simulink model "Randomized_Blending_kalman_filters"  (R2018a)
settings: Solver=ode45  StartTime=0.0  StopTime=35  FixedStep=0.05  MaxStep=0.06  RelTol=1e-3  EnableMultiTasking=on
model workspace (MAT data in the model file):
  MCOS : class17 (value not decoded)
undefined symbols (not defined in the file or in its folder): altitude_error, Continuous, error1, error2, error3, error4, fault_time, IC, quadModel, Time
libraries: simulink x5, ctrlSharedLib x4
(part 2 of 2)

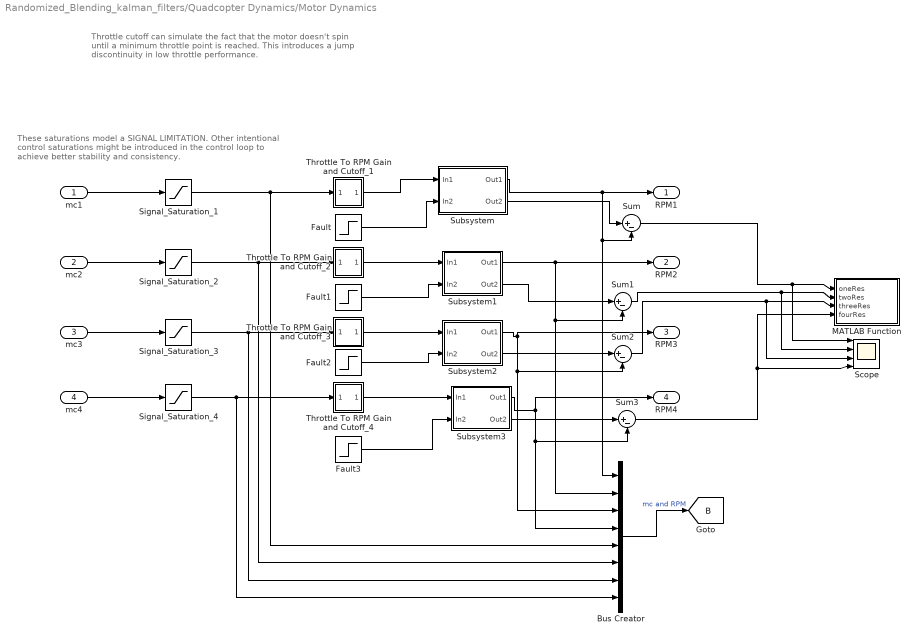
== system Randomized_Blending_kalman_filters/Quadcopter Dynamics/Motor Dynamics ==
  note: Throttle cutoff can simulate the fact that the motor doesn't
      | spin until a minimum throttle point is reached. This introduces
      | a jump discontinuity in low throttle performance.
  note: These saturations model a SIGNAL LIMITATION.
      | Other intentional control saturations might be introduced in the
      | control loop to achieve better stability and consistency.
  mc1 : Inport
  mc2 : Inport  Port=2
  mc3 : Inport  Port=3
  mc4 : Inport  Port=4
  Bus Creator : BusCreator  Inputs=8
  Fault : Step  Time=fault_time  After=error1  SampleTime=0
  Fault1 : Step  Time=fault_time  After=error2  SampleTime=0
  Fault2 : Step  Time=fault_time  After=error3  SampleTime=0
  Fault3 : Step  Time=fault_time  After=error4  SampleTime=0
  MATLAB Function : MATLAB Function  TreatAsAtomicUnit=on
  Scope : Scope  NumInputPorts=4
  Signal_Saturation_{1..4} (4 alike) : Saturate  UpperLimit=100  LowerLimit=0
  Subsystem : Subsystem
  Subsystem1 : Subsystem
  Subsystem2 : Subsystem
  Subsystem3 : Subsystem
  Sum{,1..3} (4 alike) : Sum  Inputs=|+-
  Throttle To RPM Gain and Cutoff_1 : Subsystem
  Throttle To RPM Gain and Cutoff_2 : Subsystem
  Throttle To RPM Gain and Cutoff_3 : Subsystem
  Throttle To RPM Gain and Cutoff_4 : Subsystem
  RPM1 : Outport
  RPM2 : Outport  Port=2
  RPM3 : Outport  Port=3
  RPM4 : Outport  Port=4
  tag scope: B=global
  wires:
  mc1/1 -> Signal_Saturation_1/1
  mc4/1 -> Signal_Saturation_4/1
  mc2/1 -> Signal_Saturation_2/1
  mc3/1 -> Signal_Saturation_3/1
  Signal_Saturation_1/1 -> Bus Creator/5, Throttle To RPM Gain and Cutoff_1/1(In5)
  Signal_Saturation_2/1 -> Bus Creator/6, Throttle To RPM Gain and Cutoff_2/1(In5)
  Signal_Saturation_3/1 -> Bus Creator/7, Throttle To RPM Gain and Cutoff_3/1(In5)
  Signal_Saturation_4/1 -> Bus Creator/8, Throttle To RPM Gain and Cutoff_4/1(In5)
  Throttle To RPM Gain and Cutoff_4/1(Out5) -> Subsystem3/1(In1)
  Subsystem3/1(Out1) -> RPM4/1, Sum3/2, Bus Creator/4
  Bus Creator/1 -> [B]  "mc and RPM"
  Subsystem/1(Out1) -> Sum/2, Bus Creator/1, RPM1/1
  Throttle To RPM Gain and Cutoff_1/1(Out5) -> Subsystem/1(In1)
  Fault/1 -> Subsystem/2(In2)
  Subsystem2/1(Out1) -> Sum2/2, Bus Creator/3, RPM3/1
  Subsystem1/1(Out1) -> Sum1/2, Bus Creator/2, RPM2/1
  Throttle To RPM Gain and Cutoff_2/1(Out5) -> Subsystem1/1(In1)
  Throttle To RPM Gain and Cutoff_3/1(Out5) -> Subsystem2/1(In1)
  Fault2/1 -> Subsystem2/2(In2)
  Fault3/1 -> Subsystem3/2(In2)
  Fault1/1 -> Subsystem1/2(In2)
  Subsystem/2(Out2) -> Sum/1
  Sum/1 -> Scope/1, MATLAB Function/1(oneRes)
  Subsystem3/2(Out2) -> Sum3/1
  Subsystem2/2(Out2) -> Sum2/1
  Subsystem1/2(Out2) -> Sum1/1
  Sum3/1 -> Scope/4, MATLAB Function/4(fourRes)
  Sum2/1 -> Scope/3, MATLAB Function/3(threeRes)
  Sum1/1 -> Scope/2, MATLAB Function/2(twoRes)

== system Randomized_Blending_kalman_filters/Quadcopter Dynamics/Motor Dynamics/Subsystem ==
  note: kalman filter
  note: Multiplicitive Fault
  In1 : Inport
  In2 : Inport  Port=2
  Kalman Filter : ctrlSharedLib/Kalman Filter  TimeDomain=Continuous-Time  UseCurrentEstimator=on  ModelSource=Individual A, B, C, D matrices  ModelSourceVariable=quadcopterDynamicsSFunction  A=-1/quadModel.T  B=1  C=1/quadModel.T  D=0  NumberOfStates=1  NumberOfInputs=1  NumberOfOutputs=1  InitialEstimateSource=Dialog  X0=0  P0=10  UseK=off  UseGH=off  NumberOfProcessNoiseInputs=1  G=1  TimeInvariantG=on  H=0  TimeInvariantH=on  Q=0.05  TimeInvariantQ=on  R=1  TimeInvariantR=on  N=0  TimeInvariantN=on  AddInputPort=on  AddEnablePort=off  OutputEstimatedY=on  OutputP=off  Ts=-1
      settings: SourceProductBaseCode=CT
  MATLAB Function : MATLAB Function  TreatAsAtomicUnit=on
  Motor_Dynamics_1 : StateSpace  A=-1/quadModel.T  C=1/quadModel.T  D=0  InitialCondition=IC.w1*quadModel.T
  Scope : Scope
  Out1 : Outport
  Out2 : Outport  Port=2
  wires:
  In1/1 -> Kalman Filter/1, Motor_Dynamics_1/1
  MATLAB Function/1(rotor_speed) -> Out1/1, Kalman Filter/2
  In2/1 -> MATLAB Function/1(fault)
  Motor_Dynamics_1/1 -> MATLAB Function/2(nominal_model_input)
  Kalman Filter/2 -> Scope/1, Out2/1

== system Randomized_Blending_kalman_filters/Quadcopter Dynamics/Motor Dynamics/Subsystem1 ==
  In1 : Inport
  In2 : Inport  Port=2
  Kalman Filter : ctrlSharedLib/Kalman Filter  TimeDomain=Continuous-Time  UseCurrentEstimator=on  ModelSource=Individual A, B, C, D matrices  ModelSourceVariable=quadcopterDynamicsSFunction  A=-1/quadModel.T  B=1  C=1/quadModel.T  D=0  NumberOfStates=1  NumberOfInputs=1  NumberOfOutputs=1  InitialEstimateSource=Dialog  X0=0  P0=10  UseK=off  UseGH=off  NumberOfProcessNoiseInputs=1  G=1  TimeInvariantG=on  H=0  TimeInvariantH=on  Q=0.05  TimeInvariantQ=on  R=1  TimeInvariantR=on  N=0  TimeInvariantN=on  AddInputPort=on  AddEnablePort=off  OutputEstimatedY=on  OutputP=off  Ts=-1
      settings: SourceProductBaseCode=CT
  MATLAB Function : MATLAB Function  TreatAsAtomicUnit=on
  "Motor_Dynamics_2 " : StateSpace  A=-1/quadModel.T  C=1/quadModel.T  D=0  InitialCondition=IC.w1*quadModel.T
  Out1 : Outport
  Out2 : Outport  Port=2
  wires:
  In1/1 -> "Motor_Dynamics_2 "/1, Kalman Filter/1
  MATLAB Function/1(rotor_speed) -> Kalman Filter/2, Out1/1
  In2/1 -> MATLAB Function/1(fault)
  "Motor_Dynamics_2 "/1 -> MATLAB Function/2(nominal_modal_input)
  Kalman Filter/2 -> Out2/1

== system Randomized_Blending_kalman_filters/Quadcopter Dynamics/Motor Dynamics/Subsystem2 ==
  In1 : Inport
  In2 : Inport  Port=2
  Kalman Filter : ctrlSharedLib/Kalman Filter  TimeDomain=Continuous-Time  UseCurrentEstimator=on  ModelSource=Individual A, B, C, D matrices  ModelSourceVariable=quadcopterDynamicsSFunction  A=-1/quadModel.T  B=1  C=1/quadModel.T  D=0  NumberOfStates=1  NumberOfInputs=1  NumberOfOutputs=1  InitialEstimateSource=Dialog  X0=0  P0=10  UseK=off  UseGH=off  NumberOfProcessNoiseInputs=1  G=1  TimeInvariantG=on  H=0  TimeInvariantH=on  Q=0.05  TimeInvariantQ=on  R=1  TimeInvariantR=on  N=0  TimeInvariantN=on  AddInputPort=on  AddEnablePort=off  OutputEstimatedY=on  OutputP=off  Ts=-1
      settings: SourceProductBaseCode=CT
  MATLAB Function : MATLAB Function  TreatAsAtomicUnit=on
  "Motor_Dynamics_3 " : StateSpace  A=-1/quadModel.T  C=1/quadModel.T  D=0  InitialCondition=IC.w1*quadModel.T
  Out1 : Outport
  Out2 : Outport  Port=2
  wires:
  In1/1 -> "Motor_Dynamics_3 "/1, Kalman Filter/1
  MATLAB Function/1(rotor_speed) -> Kalman Filter/2, Out1/1
  In2/1 -> MATLAB Function/1(fault)
  "Motor_Dynamics_3 "/1 -> MATLAB Function/2(nominal_modal_input)
  Kalman Filter/2 -> Out2/1

== system Randomized_Blending_kalman_filters/Quadcopter Dynamics/Motor Dynamics/Subsystem3 ==
  In1 : Inport
  In2 : Inport  Port=2
  Kalman Filter : ctrlSharedLib/Kalman Filter  TimeDomain=Continuous-Time  UseCurrentEstimator=on  ModelSource=Individual A, B, C, D matrices  ModelSourceVariable=quadcopterDynamicsSFunction  A=-1/quadModel.T  B=1  C=1/quadModel.T  D=0  NumberOfStates=1  NumberOfInputs=1  NumberOfOutputs=1  InitialEstimateSource=Dialog  X0=0  P0=10  UseK=off  UseGH=off  NumberOfProcessNoiseInputs=1  G=1  TimeInvariantG=on  H=0  TimeInvariantH=on  Q=0.05  TimeInvariantQ=on  R=1  TimeInvariantR=on  N=0  TimeInvariantN=on  AddInputPort=on  AddEnablePort=off  OutputEstimatedY=on  OutputP=off  Ts=-1
      settings: SourceProductBaseCode=CT
  MATLAB Function : MATLAB Function  TreatAsAtomicUnit=on
  "Motor_Dynamics_4 " : StateSpace  A=-1/quadModel.T  C=1/quadModel.T  D=0  InitialCondition=IC.w1*quadModel.T
  Out1 : Outport
  Out2 : Outport  Port=2
  wires:
  In1/1 -> Kalman Filter/1, "Motor_Dynamics_4 "/1
  MATLAB Function/1(rotor_speed) -> Kalman Filter/2, Out1/1
  In2/1 -> MATLAB Function/1(fault)
  "Motor_Dynamics_4 "/1 -> MATLAB Function/2(nominal_modal_input)
  Kalman Filter/2 -> Out2/1

== system Randomized_Blending_kalman_filters/Quadcopter Dynamics/Motor Dynamics/Throttle To RPM Gain and Cutoff_1 ==
  note: minThr should be a quad.mat value
  note: This gain should be a quad.mat value
  note: This constant should be a quad.mat value
  note: Output equals linearly scaled RPM
      | for given throttle input if throttle input >=Throttle Cuttoff (minThr)
      | else output is zero.
  In5 : Inport
  Constant : Constant  Value=quadModel.b
  Gain : Gain  Gain=quadModel.cr
  Minimum Throttle Cutoff : simulink/Logic and Bit Operations/Compare To Constant  relop=>=  const=quadModel.minThr  OutDataTypeStr=uint8
  Product : Product
  Sum1 : Sum  Inputs=++|
  Out5 : Outport
  wires:
  Minimum Throttle Cutoff/1 -> Product/2
  Product/1 -> Out5/1
  In5/1 -> Gain/1, Minimum Throttle Cutoff/1
  Gain/1 -> Sum1/2
  Sum1/1 -> Product/1
  Constant/1 -> Sum1/1

== system Randomized_Blending_kalman_filters/Quadcopter Dynamics/Motor Dynamics/Throttle To RPM Gain and Cutoff_2 ==
  note: minThr should be a quad.mat value
  note: This gain should be a quad.mat value
  note: This constant should be a quad.mat value
  note: Output equals linearly scaled RPM
      | for given throttle input if throttle input >=Throttle Cuttoff (minThr)
      | else output is zero.
  In5 : Inport
  Constant : Constant  Value=quadModel.b
  Gain : Gain  Gain=quadModel.cr
  Minimum Throttle Cutoff : simulink/Logic and Bit Operations/Compare To Constant  relop=>=  const=quadModel.minThr  OutDataTypeStr=uint8
  Product : Product
  Sum1 : Sum  Inputs=++|
  Out5 : Outport
  wires:
  Minimum Throttle Cutoff/1 -> Product/2
  Product/1 -> Out5/1
  In5/1 -> Gain/1, Minimum Throttle Cutoff/1
  Gain/1 -> Sum1/2
  Sum1/1 -> Product/1
  Constant/1 -> Sum1/1

== system Randomized_Blending_kalman_filters/Quadcopter Dynamics/Motor Dynamics/Throttle To RPM Gain and Cutoff_3 ==
  note: minThr should be a quad.mat value
  note: This gain should be a quad.mat value
  note: This constant should be a quad.mat value
  note: Output equals linearly scaled RPM
      | for given throttle input if throttle input >=Throttle Cuttoff (minThr)
      | else output is zero.
  In5 : Inport
  Constant : Constant  Value=quadModel.b
  Gain : Gain  Gain=quadModel.cr
  Minimum Throttle Cutoff : simulink/Logic and Bit Operations/Compare To Constant  relop=>=  const=quadModel.minThr  OutDataTypeStr=uint8
  Product : Product
  Sum1 : Sum  Inputs=++|
  Out5 : Outport
  wires:
  Minimum Throttle Cutoff/1 -> Product/2
  Product/1 -> Out5/1
  In5/1 -> Gain/1, Minimum Throttle Cutoff/1
  Gain/1 -> Sum1/2
  Sum1/1 -> Product/1
  Constant/1 -> Sum1/1

== system Randomized_Blending_kalman_filters/Quadcopter Dynamics/Motor Dynamics/Throttle To RPM Gain and Cutoff_4 ==
  note: minThr should be a quad.mat value
  note: This gain should be a quad.mat value
  note: This constant should be a quad.mat value
  note: Output equals linearly scaled RPM
      | for given throttle input if throttle input >=Throttle Cuttoff (minThr)
      | else output is zero.
  In5 : Inport
  Constant : Constant  Value=quadModel.b
  Gain : Gain  Gain=quadModel.cr
  Minimum Throttle Cutoff : simulink/Logic and Bit Operations/Compare To Constant  relop=>=  const=quadModel.minThr  OutDataTypeStr=uint8
  Product : Product
  Sum1 : Sum  Inputs=++|
  Out5 : Outport
  wires:
  Minimum Throttle Cutoff/1 -> Product/2
  Product/1 -> Out5/1
  In5/1 -> Gain/1, Minimum Throttle Cutoff/1
  Gain/1 -> Sum1/2
  Sum1/1 -> Product/1
  Constant/1 -> Sum1/1

== matlab function Randomized_Blending_kalman_filters/Quadcopter Dynamics/Motor Dynamics/Subsystem/MATLAB Function ==
  data: fault input; nominal_model_input input; rotor_speed output
function rotor_speed = fcn(fault, nominal_model_input)

rotor_speed =(nominal_model_input* (1-fault));

end

== matlab function Randomized_Blending_kalman_filters/Attitude Controller/blending  ==
  data: mode input; control_signal output; portion input; fault_controller input; nominal_controller input; wind_controller input
function control_signal = blending(mode , portion , fault_controller, nominal_controller, wind_controller)


if(mode == 1)
    fault_part = (fault_controller * portion);
    nominal_portion = 1-portion;
    nominal_part = nominal_controller * nominal_portion;
    control_signal = fault_part + nominal_part;
elseif(mode == 2)
    wind_part = (wind_controller * portion);
    nominal_portion = 1-portion;
    nominal_part = nominal_controller * nominal_portion;
    control_signal = wind_part + nominal_part;
elseif(mode == 3)
    fault_part = (fault_controller * (portion/2));
    nominal_portion = 1-portion;
    wind_part = wind_controller * (portion/2);
    nominal_part = nominal_controller * nominal_portion;
    control_signal = nominal_part + wind_part + fault_part;
else
    control_signal = nominal_controller;
end

== matlab function Randomized_Blending_kalman_filters/Quadcopter Dynamics/Motor Dynamics/Subsystem1/MATLAB Function ==
  data: fault input; nominal_modal_input input; rotor_speed output
function rotor_speed = fcn(  fault, nominal_modal_input)


rotor_speed =  (nominal_modal_input* (1-fault));

end

== matlab function Randomized_Blending_kalman_filters/Position Controller/MATLAB Function ==
  settings: updateMethod=DISCRETE
  data: y_error input; x_error input; max_error_signal data_store_memory; count data_store_memory; time input; prevTime data_store_memory
function fcn(y_error,x_error,time)
global prevTime;
global max_error_signal;
global count;
%if(abs(y_error) + abs(x_error) > max_error_signal)
if(prevTime+0.1 < time)
    max_error_signal = max_error_signal + abs(y_error) + abs(x_error);
    count =count +1;
    %disp(count);
    prevTime = time;
end
end

== matlab function Randomized_Blending_kalman_filters/Quadcopter Dynamics/Motor Dynamics/Subsystem2/MATLAB Function ==
  data: fault input; nominal_modal_input input; rotor_speed output
function rotor_speed = fcn(  fault, nominal_modal_input)


rotor_speed =  (nominal_modal_input* (1-fault));

end

== matlab function Randomized_Blending_kalman_filters/Quadcopter Dynamics/Motor Dynamics/Subsystem3/MATLAB Function ==
  data: fault input; nominal_modal_input input; rotor_speed output
function rotor_speed = fcn(  fault, nominal_modal_input)


rotor_speed =  (nominal_modal_input* (1-fault));

end

== matlab function Randomized_Blending_kalman_filters/Attitude Controller/blending 1 ==
  data: mode input; control_signal output; portion input; fault_controller input; nominal_controller input; wind_controller input
function control_signal = blending(mode , portion , fault_controller, nominal_controller, wind_controller)


if(mode == 1)
    fault_part = (fault_controller * portion);
    nominal_portion = 1-portion;
    nominal_part = nominal_controller * nominal_portion;
    control_signal = fault_part + nominal_part;
elseif(mode == 2)
    wind_part = (wind_controller * portion);
    nominal_portion = 1-portion;
    nominal_part = nominal_controller * nominal_portion;
    control_signal = wind_part + nominal_part;
elseif(mode == 3)
    fault_part = (fault_controller * (portion/2));
    nominal_portion = 1-portion;
    wind_part = wind_controller * (portion/2);
    nominal_part = nominal_controller * nominal_portion;
    control_signal = nominal_part + wind_part + fault_part;
else
    control_signal = nominal_controller;
end

== matlab function Randomized_Blending_kalman_filters/Attitude Controller/blending 2 ==
  data: mode input; control_signal output; portion input; fault_controller input; nominal_controller input; wind_controller input
function control_signal = blending(mode , portion , fault_controller, nominal_controller, wind_controller)


if(mode == 1)
    fault_part = (fault_controller * portion);
    nominal_portion = 1-portion;
    nominal_part = nominal_controller * nominal_portion;
    control_signal = fault_part + nominal_part;
elseif(mode == 2)
    wind_part = (wind_controller * portion);
    nominal_portion = 1-portion;
    nominal_part = nominal_controller * nominal_portion;
    control_signal = wind_part + nominal_part;
elseif(mode == 3)
    fault_part = (fault_controller * (portion/2));
    nominal_portion = 1-portion;
    wind_part = wind_controller * (portion/2);
    nominal_part = nominal_controller * nominal_portion;
    control_signal = nominal_part + wind_part + fault_part;
else
    control_signal = nominal_controller;
end

== matlab function Randomized_Blending_kalman_filters/Attitude Controller/High Level Randomised Algorithm ==
  settings: updateMethod=DISCRETE
  data: x_error input; y_error input; Phi output; Theta output; Psi output; previousTime data_store_memory; blend data_store_memory; time input; Phi_blend data_store_memory; Theta_blend data_store_memory; Psi_blend data_store_memory; errors data_store_memory; rate_of_change data_store_memory; rate output; current_error output; prev_rate_of_change data_store_memory; fault_est data_store_memory; fault output
function [Phi, Theta, Psi, rate, current_error, fault] = fcn(x_error, y_error, time)
%global lookup_table;
global previousTime;
global errors;
%current_error_index = (current_error*1000) +1;
global Phi_blend;
global Theta_blend;
global Psi_blend;
global rate_of_change;
global prev_rate_of_change;

global fault_est;

%distance to desired location
current_error = sqrt(x_error^2 + y_error^2);

%previous distance and current distance
if(time > previousTime(5))
    errors(1) = errors(2);
    errors(2) = errors(3);
    errors(3) = errors(4);
    errors(4) = errors(5);
    errors(5) = current_error;

    previousTime(1) = previousTime(2);
    previousTime(2) = previousTime(3);
    previousTime(3) = previousTime(4);
    previousTime(4) = previousTime(5);
    previousTime(5) = time;

    curve = polyfit(previousTime,errors , 4);
    derivative = polyder(curve);
    prev_rate_of_change = rate_of_change;
    rate_of_change =  polyval(derivative,time);
    %disp('--------------');
    %disp(time);
    %disp(rate_of_change);
    %disp(abs(current_error));
    rate = rate_of_change;
    
else
    rate = rate_of_change;
end
%if(rate_of_change > 0.3 && prev_rate_of_change > 0.3 && current_error > 0.3)

if(time > 15 )
    %blend = 0;
    %blend = 1;
    %blend = rand();
    %Phi = blend;
    %Theta= blend;
    %Psi = blend;
    %(BOTH WIND AND ROTOR)
    %fault = 3;
    % Phi_blend = blend;
    %Theta_blend =blend;
    %Psi_blend = blend;
    Phi = Phi_blend;
    Theta= Theta_blend;
    Psi = Psi_blend;
    fault = 1;
    
%no rotor fault but external disturbance 
elseif( time > 17 && rate_of_change > 0.2 && prev_rate_of_change > 0.2 )
    blend = rand();
    Phi = blend;
    Theta= blend;
    Psi = blend;
    fault = 1;
    %blend = 1;
    %
    %blend = 0;
    %Phi = blend;
    %Theta= blend;
    %Psi = blend;
    %(WIND)
    %fault = 2;
    %Phi_blend = blend;
    %Theta_blend =blend;
    %Psi_blend = blend;

%rotor fault and external disturbance
%elseif(fault_est == 1)
    %blend = rand();
    %blend = 1;
   % blend = 0;
   % Phi = blend;
   % Theta= blend;
    %Psi = blend;
    %(ROTOR)
    %fault = 1;
   % Phi_blend = blend;
    %Theta_blend =blend;
    %Psi_blend = blend;
    %Phi = Phi_blend;
    %Theta= Theta_blend;
    %Psi = Psi_blend;
    %fault = 1;
else
    %(No fault)
    blend = 0;
    %Phi = blend;
    %Theta= blend;
    %Psi = blend;
    %blend = 0;
    Phi = blend;
    Theta= blend;
    Psi = blend;
    fault = 1;
end

== matlab function Randomized_Blending_kalman_filters/Position Controller/MATLAB Function1 ==
  settings: updateMethod=DISCRETE
  data: alt_diff input; y output; altitude_error data_store_memory; time input; PrevTime2 data_store_memory
function y = fcn(alt_diff, time)
global altitude_error;
global PrevTime2;

if(PrevTime2+0.1 < time)
    altitude_error = altitude_error + abs(alt_diff);

    y = altitude_error;
    PrevTime2 = time;
else
    y = altitude_error;
end

== matlab function Randomized_Blending_kalman_filters/Quadcopter Dynamics/Motor Dynamics/MATLAB Function ==
  settings: updateMethod=DISCRETE
  data: oneRes input; twoRes input; threeRes input; fourRes input; fault_est data_store_memory
function fcn(oneRes, twoRes, threeRes, fourRes)
global fault_est;
maxRes = max([oneRes twoRes threeRes fourRes]);
%threshold in rpm 
RPMthreshold = 50;

if(maxRes > RPMthreshold)
    fault_est = 1;
else
    fault_est = 0;
end
